simulink model "TestVerticalThrustComp"  (R2018b)
settings: Solver=VariableStepAuto  StartTime=0.0  StopTime=10.0  RelTol=1e-3
libraries: QuaternionLibrary x15, simulink_extras x1
settings Model: Creator=jban039  LastModifiedBy=jban039

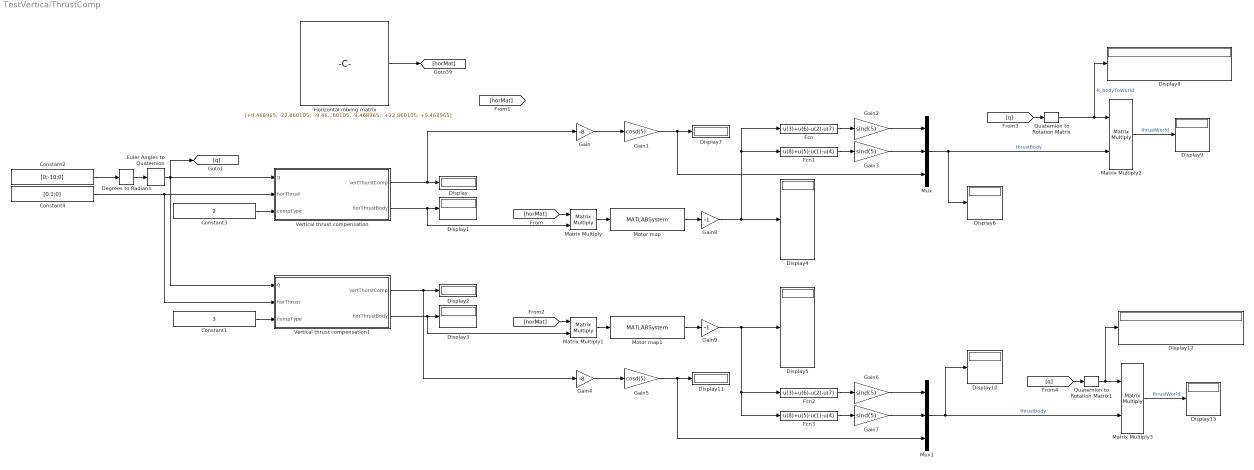
== system TestVerticalThrustComp ==
  Constant1 : Constant  Value=3
  Constant2 : Constant  Value=[0;-10;0]
  Constant3 : Constant  Value=2
  Constant4 : Constant  Value=[0.1;0]
  Degrees to Radians : simulink_extras/Transformations/Degrees to Radians
  Display{,1..13} (14 alike) : Display
  Euler Angles to Quaternion : QuaternionLibrary/Euler Angles to Quaternion
  Fcn : Fcn  Expr=u(3)+u(6)-u(2)-u(7)
  Fcn1 : Fcn  Expr=u(8)+u(5)-u(1)-u(4)
  Fcn2 : Fcn  Expr=u(3)+u(6)-u(2)-u(7)
  Fcn3 : Fcn  Expr=u(8)+u(5)-u(1)-u(4)
  Gain : Gain  Gain=-8
  Gain1 : Gain  Gain=cosd(5)
  Gain{2..3,6..7} (4 alike) : Gain  Gain=sind(5)
  Gain4 : Gain  Gain=-8
  Gain5 : Gain  Gain=cosd(5)
  Gain8 : Gain  Gain=-1
  Gain9 : Gain  Gain=-1
  Horizontal mixing matrix : Constant  Value=|
      | [+9.468965, -22.860105;
      |  -9.468965, +22.860105;
      |  -22.860105, +9.468965;
      |  -9.468965, -22.860105;
      |  +9.468965, +22.860105;
      |  +22.860105, -9.468965;
      |  -22.860105, -9.468965;
      |  +22.860105, +9.468965]
  Matrix Multiply{,1..3} (4 alike) : Product  Multiplication=Matrix(*)
  Motor map : MATLABSystem  System=MotorMap  airframeConfig=5  SimulateUsing=Code generation
      mask Type: MotorMap
      mask Display:
      | disp(['MOTOR' char(10) 'MAP' char(10) 'octa_x']);
      | port_label('input',1,'px4PWM');
      | port_label('output',1,'simPWM');
  Motor map1 : MATLABSystem  System=MotorMap  airframeConfig=5  SimulateUsing=Code generation
      mask Type: MotorMap
      mask Display:
      | disp(['MOTOR' char(10) 'MAP' char(10) 'octa_x']);
      | port_label('input',1,'px4PWM');
      | port_label('output',1,'simPWM');
  Mux : Mux  Inputs=3
  Mux1 : Mux  Inputs=3
  Quaternion to Rotation Matrix : QuaternionLibrary/Quaternion to Rotation Matrix
  Quaternion to Rotation Matrix1 : QuaternionLibrary/Quaternion to Rotation Matrix
  Vertical thrust compensation : Subsystem
  Vertical thrust compensation1 : Subsystem
  wires:
  Constant3/1 -> Vertical thrust compensation/3(compType)
  Constant1/1 -> Vertical thrust compensation1/3(compType)
  Constant2/1 -> Degrees to Radians/1
  Constant4/1 -> Vertical thrust compensation1/2("horThrust "), Vertical thrust compensation/2("horThrust ")
  Euler Angles to Quaternion/1 -> [q], Vertical thrust compensation1/1("q "), Vertical thrust compensation/1("q ")
  Vertical thrust compensation/1(" vertThurstComp") -> Gain/1, Display/1
  Vertical thrust compensation/2(" horThrustBody") -> Matrix Multiply/2, Display1/1
  Horizontal mixing matrix/1 -> [horMat]
  [horMat] -> Matrix Multiply/1
  [horMat] -> Matrix Multiply1/1
  Vertical thrust compensation1/2(" horThrustBody") -> Matrix Multiply1/2, Display3/1
  Matrix Multiply/1 -> Motor map/1
  Matrix Multiply1/1 -> Motor map1/1
  Gain/1 -> Gain1/1
  Motor map/1 -> Gain8/1
  Fcn/1 -> Gain2/1
  Gain2/1 -> Mux/1
  Gain1/1 -> Mux/3, Display7/1
  Fcn1/1 -> Gain3/1
  Gain3/1 -> Mux/2
  Quaternion to Rotation Matrix/1 -> Display8/1, Matrix Multiply2/1  "R_bodyToWorld"
  Mux/1 -> Matrix Multiply2/2, Display6/1  "thrustBody"
  [q] -> Quaternion to Rotation Matrix/1
  Matrix Multiply2/1 -> Display9/1  "thrustWorld"
  Degrees to Radians/1 -> Euler Angles to Quaternion/1
  Matrix Multiply3/1 -> Display13/1  "thrustWorld"
  [q] -> Quaternion to Rotation Matrix1/1
  Mux1/1 -> Display10/1, Matrix Multiply3/2  "thrustBody"
  Quaternion to Rotation Matrix1/1 -> Matrix Multiply3/1, Display12/1
  Gain7/1 -> Mux1/2
  Fcn3/1 -> Gain7/1
  Gain5/1 -> Display11/1, Mux1/3
  Gain6/1 -> Mux1/1
  Fcn2/1 -> Gain6/1
  Motor map1/1 -> Gain9/1
  Gain4/1 -> Gain5/1
  Vertical thrust compensation1/1(" vertThurstComp") -> Gain4/1, Display2/1
  Gain8/1 -> Fcn/1, Fcn1/1, Display4/1
  Gain9/1 -> Fcn3/1, Fcn2/1, Display5/1

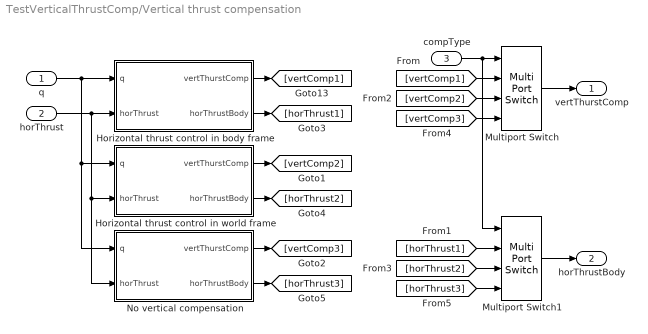
== system TestVerticalThrustComp/Vertical thrust compensation ==
  "q " : Inport
  "horThrust " : Inport  Port=2
  compType : Inport  Port=3
  Horizontal thrust control in body frame : Subsystem  VariantControl=HorThrustBodyFrame
  Horizontal thrust control in world frame : Subsystem  VariantControl=HorThrustWorldFrame
  Multiport Switch : MultiPortSwitch
  Multiport Switch1 : MultiPortSwitch
  No vertical compensation : Subsystem  VariantControl=HorThrustNoVertComp
  " vertThurstComp" : Outport
  " horThrustBody" : Outport  Port=2
  wires:
  [horThrust1] -> Multiport Switch1/2
  [horThrust2] -> Multiport Switch1/3
  [horThrust3] -> Multiport Switch1/4
  [vertComp3] -> Multiport Switch/4
  [vertComp2] -> Multiport Switch/3
  [vertComp1] -> Multiport Switch/2
  No vertical compensation/2(" horThrustBody") -> [horThrust3]
  Horizontal thrust control in world frame/2(" horThrustBody") -> [horThrust2]
  Horizontal thrust control in body frame/2(horThrustBody) -> [horThrust1]
  No vertical compensation/1(" vertThurstComp") -> [vertComp3]
  Horizontal thrust control in world frame/1(" vertThurstComp") -> [vertComp2]
  Horizontal thrust control in body frame/1(vertThurstComp) -> [vertComp1]
  compType/1 -> Multiport Switch/1, Multiport Switch1/1
  Multiport Switch1/1 -> " horThrustBody"/1
  Multiport Switch/1 -> " vertThurstComp"/1
  "horThrust "/1 -> Horizontal thrust control in body frame/2(horThrust), No vertical compensation/2("horThrust "), Horizontal thrust control in world frame/2("horThrust ")
  "q "/1 -> Horizontal thrust control in body frame/1(q), Horizontal thrust control in world frame/1("q "), No vertical compensation/1("q ")

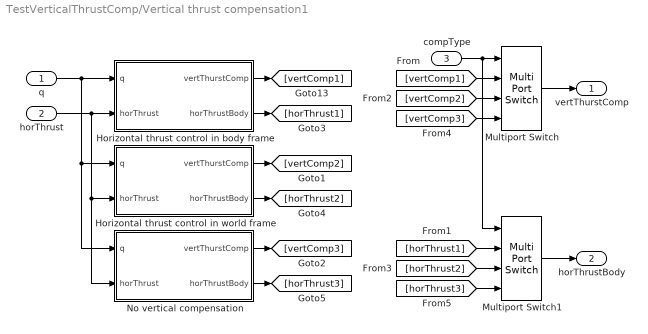
== system TestVerticalThrustComp/Vertical thrust compensation1 ==
  "q " : Inport
  "horThrust " : Inport  Port=2
  compType : Inport  Port=3
  Horizontal thrust control in body frame : Subsystem  VariantControl=HorThrustBodyFrame
  Horizontal thrust control in world frame : Subsystem  VariantControl=HorThrustWorldFrame
  Multiport Switch : MultiPortSwitch
  Multiport Switch1 : MultiPortSwitch
  No vertical compensation : Subsystem  VariantControl=HorThrustNoVertComp
  " vertThurstComp" : Outport
  " horThrustBody" : Outport  Port=2
  wires:
  "q "/1 -> No vertical compensation/1("q "), Horizontal thrust control in world frame/1("q "), Horizontal thrust control in body frame/1(q)
  "horThrust "/1 -> Horizontal thrust control in world frame/2("horThrust "), No vertical compensation/2("horThrust "), Horizontal thrust control in body frame/2(horThrust)
  Multiport Switch/1 -> " vertThurstComp"/1
  Multiport Switch1/1 -> " horThrustBody"/1
  compType/1 -> Multiport Switch1/1, Multiport Switch/1
  Horizontal thrust control in body frame/1(vertThurstComp) -> [vertComp1]
  Horizontal thrust control in world frame/1(" vertThurstComp") -> [vertComp2]
  No vertical compensation/1(" vertThurstComp") -> [vertComp3]
  Horizontal thrust control in body frame/2(horThrustBody) -> [horThrust1]
  Horizontal thrust control in world frame/2(" horThrustBody") -> [horThrust2]
  No vertical compensation/2(" horThrustBody") -> [horThrust3]
  [vertComp1] -> Multiport Switch/2
  [vertComp2] -> Multiport Switch/3
  [vertComp3] -> Multiport Switch/4
  [horThrust3] -> Multiport Switch1/4
  [horThrust2] -> Multiport Switch1/3
  [horThrust1] -> Multiport Switch1/2

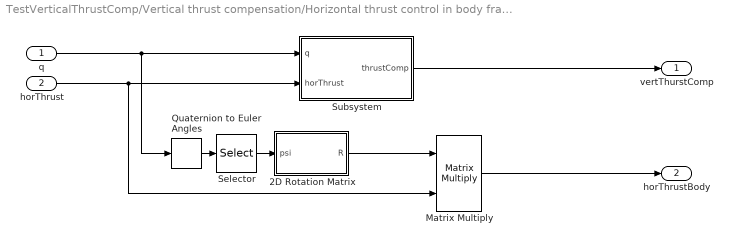
== system TestVerticalThrustComp/Vertical thrust compensation/Horizontal thrust control in body frame ==
  q : Inport
  horThrust : Inport  Port=2
  2D Rotation Matrix : Subsystem
  Matrix Multiply : Product  Multiplication=Matrix(*)
  Quaternion to Euler Angles : QuaternionLibrary/Quaternion to Euler Angles
  Selector : Selector  InputPortWidth=3  IndexOptions=Index vector (dialog)  Indices=3  OutputSizes=1
  Subsystem : Subsystem
  vertThurstComp : Outport
  horThrustBody : Outport  Port=2
  wires:
  Matrix Multiply/1 -> horThrustBody/1
  2D Rotation Matrix/1(R) -> Matrix Multiply/1
  Selector/1 -> 2D Rotation Matrix/1(psi)
  Subsystem/1(thrustComp) -> vertThurstComp/1
  Quaternion to Euler Angles/1 -> Selector/1
  q/1 -> Subsystem/1(q), Quaternion to Euler Angles/1
  horThrust/1 -> Subsystem/2(horThrust), Matrix Multiply/2

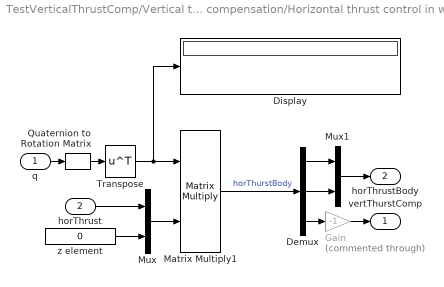
== system TestVerticalThrustComp/Vertical thrust compensation/Horizontal thrust control in world frame ==
  "q " : Inport
  "horThrust " : Inport  Port=2
  Demux : Demux  Outputs=3
  Display : Display
  Gain : Gain  Commented=through  Gain=-1
  Matrix Multiply1 : Product  Multiplication=Matrix(*)
  Mux : Mux  Inputs=2
  Mux1 : Mux  Inputs=2
  Quaternion to Rotation Matrix : QuaternionLibrary/Quaternion to Rotation Matrix
  Transpose : Math  Operator=transpose  SaturateOnIntegerOverflow=on
  z element : Constant  Value=0
  " vertThurstComp" : Outport
  " horThrustBody" : Outport  Port=2
  wires:
  Gain/1 -> " vertThurstComp"/1
  Demux/3 -> Gain/1
  Mux1/1 -> " horThrustBody"/1
  Demux/1 -> Mux1/1
  Demux/2 -> Mux1/2
  Matrix Multiply1/1 -> Demux/1  "horThurstBody"
  Transpose/1 -> Display/1, Matrix Multiply1/1
  "q "/1 -> Quaternion to Rotation Matrix/1
  "horThrust "/1 -> Mux/1
  z element/1 -> Mux/2
  Mux/1 -> Matrix Multiply1/2
  Quaternion to Rotation Matrix/1 -> Transpose/1

== system TestVerticalThrustComp/Vertical thrust compensation/No vertical compensation ==
  "q " : Inport
  "horThrust " : Inport  Port=2
  2D Rotation Matrix : Subsystem
  Ground : Ground
  Matrix Multiply : Product  Multiplication=Matrix(*)
  Quaternion to Euler Angles : QuaternionLibrary/Quaternion to Euler Angles
  Selector : Selector  InputPortWidth=3  IndexOptions=Index vector (dialog)  Indices=3  OutputSizes=1
  " vertThurstComp" : Outport
  " horThrustBody" : Outport  Port=2
  wires:
  "horThrust "/1 -> Matrix Multiply/2
  Quaternion to Euler Angles/1 -> Selector/1
  Selector/1 -> 2D Rotation Matrix/1(psi)
  "q "/1 -> Quaternion to Euler Angles/1
  2D Rotation Matrix/1(R) -> Matrix Multiply/1
  Ground/1 -> " vertThurstComp"/1
  Matrix Multiply/1 -> " horThrustBody"/1

== system TestVerticalThrustComp/Vertical thrust compensation1/Horizontal thrust control in body frame ==
  q : Inport
  horThrust : Inport  Port=2
  2D Rotation Matrix : Subsystem
  Matrix Multiply : Product  Multiplication=Matrix(*)
  Quaternion to Euler Angles : QuaternionLibrary/Quaternion to Euler Angles
  Selector : Selector  InputPortWidth=3  IndexOptions=Index vector (dialog)  Indices=3  OutputSizes=1
  Subsystem : Subsystem
  vertThurstComp : Outport
  horThrustBody : Outport  Port=2
  wires:
  horThrust/1 -> Matrix Multiply/2, Subsystem/2(horThrust)
  q/1 -> Quaternion to Euler Angles/1, Subsystem/1(q)
  Quaternion to Euler Angles/1 -> Selector/1
  Subsystem/1(thrustComp) -> vertThurstComp/1
  Selector/1 -> 2D Rotation Matrix/1(psi)
  2D Rotation Matrix/1(R) -> Matrix Multiply/1
  Matrix Multiply/1 -> horThrustBody/1

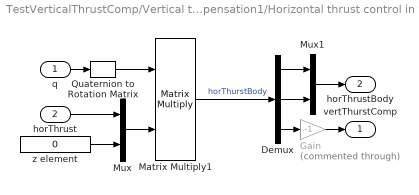
== system TestVerticalThrustComp/Vertical thrust compensation1/Horizontal thrust control in world frame ==
  "q " : Inport
  "horThrust " : Inport  Port=2
  Demux : Demux  Outputs=3
  Gain : Gain  Commented=through  Gain=-1
  Matrix Multiply1 : Product  Multiplication=Matrix(*)
  Mux : Mux  Inputs=2
  Mux1 : Mux  Inputs=2
  Quaternion to Rotation Matrix : QuaternionLibrary/Quaternion to Rotation Matrix
  z element : Constant  Value=0
  " vertThurstComp" : Outport
  " horThrustBody" : Outport  Port=2
  wires:
  Mux/1 -> Matrix Multiply1/2
  z element/1 -> Mux/2
  "horThrust "/1 -> Mux/1
  "q "/1 -> Quaternion to Rotation Matrix/1
  Quaternion to Rotation Matrix/1 -> Matrix Multiply1/1
  Matrix Multiply1/1 -> Demux/1  "horThurstBody"
  Demux/2 -> Mux1/2
  Demux/1 -> Mux1/1
  Mux1/1 -> " horThrustBody"/1
  Demux/3 -> Gain/1
  Gain/1 -> " vertThurstComp"/1

== system TestVerticalThrustComp/Vertical thrust compensation1/No vertical compensation ==
  "q " : Inport
  "horThrust " : Inport  Port=2
  2D Rotation Matrix : Subsystem
  Ground : Ground
  Matrix Multiply : Product  Multiplication=Matrix(*)
  Quaternion to Euler Angles : QuaternionLibrary/Quaternion to Euler Angles
  Selector : Selector  InputPortWidth=3  IndexOptions=Index vector (dialog)  Indices=3  OutputSizes=1
  " vertThurstComp" : Outport
  " horThrustBody" : Outport  Port=2
  wires:
  Matrix Multiply/1 -> " horThrustBody"/1
  Ground/1 -> " vertThurstComp"/1
  2D Rotation Matrix/1(R) -> Matrix Multiply/1
  "q "/1 -> Quaternion to Euler Angles/1
  Selector/1 -> 2D Rotation Matrix/1(psi)
  Quaternion to Euler Angles/1 -> Selector/1
  "horThrust "/1 -> Matrix Multiply/2

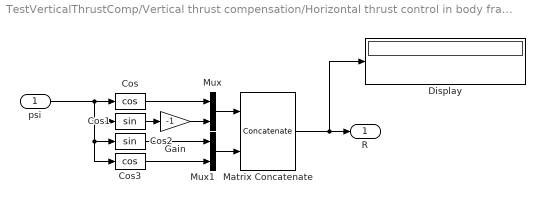
== system TestVerticalThrustComp/Vertical thrust compensation/Horizontal thrust control in body frame/2D Rotation Matrix ==
  psi : Inport
  Cos : Trigonometry  Operator=cos
  Cos1 : Trigonometry
  Cos2 : Trigonometry
  Cos3 : Trigonometry  Operator=cos
  Display : Display
  Gain : Gain  Gain=-1
  Matrix Concatenate : Concatenate  Mode=Multidimensional array  ConcatenateDimension=2
  Mux : Mux  Inputs=2
  Mux1 : Mux  Inputs=2
  R : Outport
  wires:
  psi/1 -> Cos3/1, Cos2/1, Cos1/1, Cos/1
  Matrix Concatenate/1 -> R/1, Display/1
  Mux1/1 -> Matrix Concatenate/2
  Gain/1 -> Mux/2
  Cos/1 -> Mux/1
  Cos1/1 -> Gain/1
  Mux/1 -> Matrix Concatenate/1
  Cos2/1 -> Mux1/1
  Cos3/1 -> Mux1/2

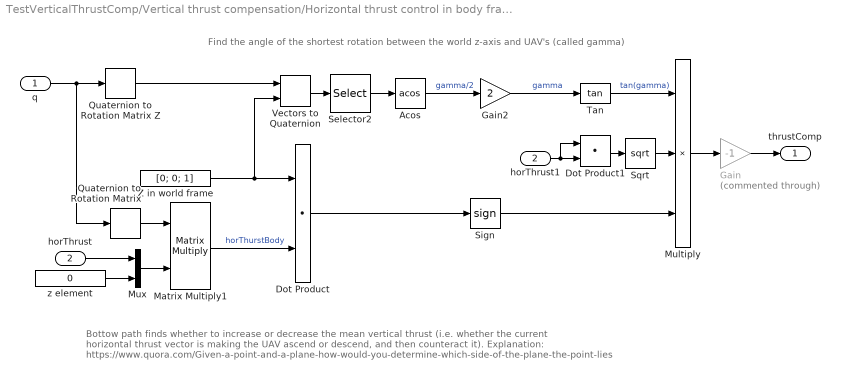
== system TestVerticalThrustComp/Vertical thrust compensation/Horizontal thrust control in body frame/Subsystem ==
  note: Bottow path finds whether to increase or decrease the mean vertical thrust (i.e. whether the current horizontal thrust vector is
      | making the UAV ascend or descend, and then counteract it).
      | Explanation: https://www.quora.com/Given-a-point-and-a-plane-how-would-you-determine-which-side-of-the-plane-the-point-lies
  note: Find the angle of the shortest rotation between the world z-axis and UAV's (called gamma)
  q : Inport
  horThrust : Inport  Port=2
  Acos : Trigonometry  Operator=acos
  Dot Product : DotProduct  InputSameDT=on  OutDataTypeStr=Inherit: Inherit via internal rule
  Dot Product1 : DotProduct  InputSameDT=on  OutDataTypeStr=Inherit: Inherit via internal rule
  Gain : Gain  Commented=through  Gain=-1
  Gain2 : Gain  Gain=2
  Matrix Multiply1 : Product  Multiplication=Matrix(*)
  Multiply : Product  Inputs=***
  Mux : Mux  Inputs=2
  Quaternion to Rotation Matrix : QuaternionLibrary/Quaternion to Rotation Matrix
  Quaternion to Rotation Matrix Z : QuaternionLibrary/Quaternion to Rotation Matrix Z
  Selector2 : Selector  InputPortWidth=4  IndexOptions=Index vector (dialog)  Indices=1  OutputSizes=1
  Sign : Signum
  Sqrt : Sqrt  SaturateOnIntegerOverflow=on
  Tan : Trigonometry  Operator=tan
  Vectors to Quaternion : QuaternionLibrary/Vectors to Quaternion
  Z in world frame : Constant  Value=[0; 0; 1]
  horThrust1 : InportShadow  Port=2
  z element : Constant  Value=0
  thrustComp : Outport
  wires:
  Gain/1 -> thrustComp/1
  Sqrt/1 -> Multiply/2
  horThrust1/1 -> Dot Product1/2, Dot Product1/1
  Dot Product1/1 -> Sqrt/1
  Tan/1 -> Multiply/1  "tan(gamma)"
  horThrust/1 -> Mux/1
  Sign/1 -> Multiply/3
  Mux/1 -> Matrix Multiply1/2
  z element/1 -> Mux/2
  Z in world frame/1 -> Dot Product/1, Vectors to Quaternion/2
  q/1 -> Quaternion to Rotation Matrix Z/1, Quaternion to Rotation Matrix/1
  Quaternion to Rotation Matrix/1 -> Matrix Multiply1/1
  Multiply/1 -> Gain/1
  Quaternion to Rotation Matrix Z/1 -> Vectors to Quaternion/1
  Gain2/1 -> Tan/1  "gamma"
  Dot Product/1 -> Sign/1
  Matrix Multiply1/1 -> Dot Product/2  "horThurstBody"
  Acos/1 -> Gain2/1  "gamma/2"
  Vectors to Quaternion/1 -> Selector2/1
  Selector2/1 -> Acos/1

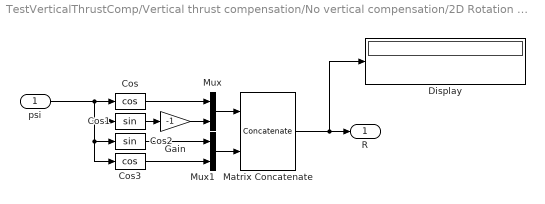
== system TestVerticalThrustComp/Vertical thrust compensation/No vertical compensation/2D Rotation Matrix ==
  psi : Inport
  Cos : Trigonometry  Operator=cos
  Cos1 : Trigonometry
  Cos2 : Trigonometry
  Cos3 : Trigonometry  Operator=cos
  Display : Display
  Gain : Gain  Gain=-1
  Matrix Concatenate : Concatenate  Mode=Multidimensional array  ConcatenateDimension=2
  Mux : Mux  Inputs=2
  Mux1 : Mux  Inputs=2
  R : Outport
  wires:
  psi/1 -> Cos3/1, Cos2/1, Cos1/1, Cos/1
  Matrix Concatenate/1 -> R/1, Display/1
  Mux1/1 -> Matrix Concatenate/2
  Gain/1 -> Mux/2
  Cos/1 -> Mux/1
  Cos1/1 -> Gain/1
  Mux/1 -> Matrix Concatenate/1
  Cos2/1 -> Mux1/1
  Cos3/1 -> Mux1/2

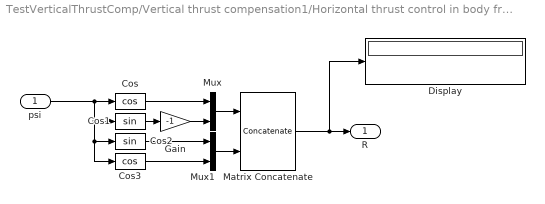
== system TestVerticalThrustComp/Vertical thrust compensation1/Horizontal thrust control in body frame/2D Rotation Matrix ==
  psi : Inport
  Cos : Trigonometry  Operator=cos
  Cos1 : Trigonometry
  Cos2 : Trigonometry
  Cos3 : Trigonometry  Operator=cos
  Display : Display
  Gain : Gain  Gain=-1
  Matrix Concatenate : Concatenate  Mode=Multidimensional array  ConcatenateDimension=2
  Mux : Mux  Inputs=2
  Mux1 : Mux  Inputs=2
  R : Outport
  wires:
  Cos3/1 -> Mux1/2
  Cos2/1 -> Mux1/1
  Mux/1 -> Matrix Concatenate/1
  Cos1/1 -> Gain/1
  Cos/1 -> Mux/1
  Gain/1 -> Mux/2
  Mux1/1 -> Matrix Concatenate/2
  Matrix Concatenate/1 -> Display/1, R/1
  psi/1 -> Cos/1, Cos1/1, Cos2/1, Cos3/1

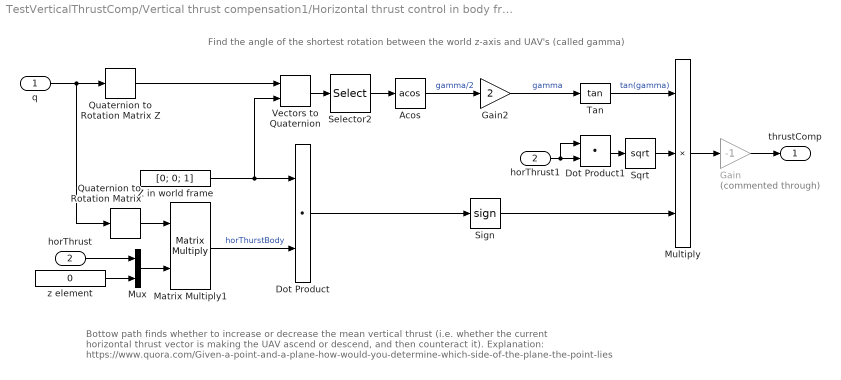
== system TestVerticalThrustComp/Vertical thrust compensation1/Horizontal thrust control in body frame/Subsystem ==
  note: Find the angle of the shortest rotation between the world z-axis and UAV's (called gamma)
  note: Bottow path finds whether to increase or decrease the mean vertical thrust (i.e. whether the current horizontal thrust vector is
      | making the UAV ascend or descend, and then counteract it).
      | Explanation: https://www.quora.com/Given-a-point-and-a-plane-how-would-you-determine-which-side-of-the-plane-the-point-lies
  q : Inport
  horThrust : Inport  Port=2
  Acos : Trigonometry  Operator=acos
  Dot Product : DotProduct  InputSameDT=on  OutDataTypeStr=Inherit: Inherit via internal rule
  Dot Product1 : DotProduct  InputSameDT=on  OutDataTypeStr=Inherit: Inherit via internal rule
  Gain : Gain  Commented=through  Gain=-1
  Gain2 : Gain  Gain=2
  Matrix Multiply1 : Product  Multiplication=Matrix(*)
  Multiply : Product  Inputs=***
  Mux : Mux  Inputs=2
  Quaternion to Rotation Matrix : QuaternionLibrary/Quaternion to Rotation Matrix
  Quaternion to Rotation Matrix Z : QuaternionLibrary/Quaternion to Rotation Matrix Z
  Selector2 : Selector  InputPortWidth=4  IndexOptions=Index vector (dialog)  Indices=1  OutputSizes=1
  Sign : Signum
  Sqrt : Sqrt  SaturateOnIntegerOverflow=on
  Tan : Trigonometry  Operator=tan
  Vectors to Quaternion : QuaternionLibrary/Vectors to Quaternion
  Z in world frame : Constant  Value=[0; 0; 1]
  horThrust1 : InportShadow  Port=2
  z element : Constant  Value=0
  thrustComp : Outport
  wires:
  Selector2/1 -> Acos/1
  Vectors to Quaternion/1 -> Selector2/1
  Acos/1 -> Gain2/1  "gamma/2"
  Matrix Multiply1/1 -> Dot Product/2  "horThurstBody"
  Dot Product/1 -> Sign/1
  Gain2/1 -> Tan/1  "gamma"
  Quaternion to Rotation Matrix Z/1 -> Vectors to Quaternion/1
  Multiply/1 -> Gain/1
  Quaternion to Rotation Matrix/1 -> Matrix Multiply1/1
  q/1 -> Quaternion to Rotation Matrix/1, Quaternion to Rotation Matrix Z/1
  Z in world frame/1 -> Vectors to Quaternion/2, Dot Product/1
  z element/1 -> Mux/2
  Mux/1 -> Matrix Multiply1/2
  Sign/1 -> Multiply/3
  horThrust/1 -> Mux/1
  Tan/1 -> Multiply/1  "tan(gamma)"
  Dot Product1/1 -> Sqrt/1
  horThrust1/1 -> Dot Product1/1, Dot Product1/2
  Sqrt/1 -> Multiply/2
  Gain/1 -> thrustComp/1

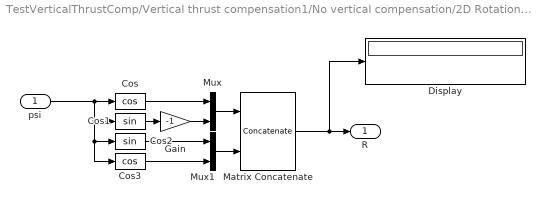
== system TestVerticalThrustComp/Vertical thrust compensation1/No vertical compensation/2D Rotation Matrix ==
  psi : Inport
  Cos : Trigonometry  Operator=cos
  Cos1 : Trigonometry
  Cos2 : Trigonometry
  Cos3 : Trigonometry  Operator=cos
  Display : Display
  Gain : Gain  Gain=-1
  Matrix Concatenate : Concatenate  Mode=Multidimensional array  ConcatenateDimension=2
  Mux : Mux  Inputs=2
  Mux1 : Mux  Inputs=2
  R : Outport
  wires:
  Cos3/1 -> Mux1/2
  Cos2/1 -> Mux1/1
  Mux/1 -> Matrix Concatenate/1
  Cos1/1 -> Gain/1
  Cos/1 -> Mux/1
  Gain/1 -> Mux/2
  Mux1/1 -> Matrix Concatenate/2
  Matrix Concatenate/1 -> Display/1, R/1
  psi/1 -> Cos/1, Cos1/1, Cos2/1, Cos3/1
